simulink model "KakmanFilterSonarExample__Simtestbench"  (R2023b)
settings: Solver=FixedStepAuto  StartTime=0.0  StopTime=Ts*(numel(sonarAlt)-1)  FixedStep=Ts  RelTol=1e-3
undefined symbols (not defined in the file): Discrete, Time, Ts
libraries: simulink x1, ctrlSharedLib x1
settings Model: Creator=leoni  LastModifiedBy=leoni

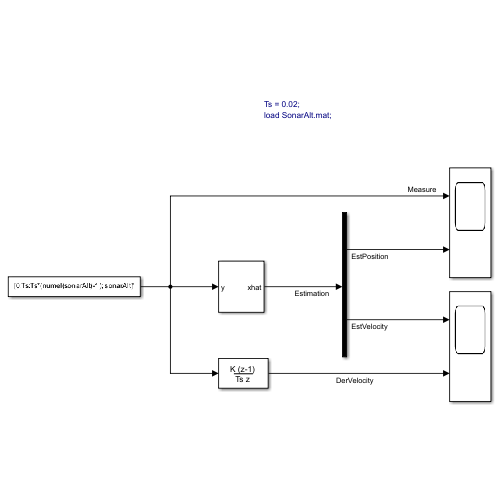
[thumbnail: Simulink's stored preview of the top-level diagram]
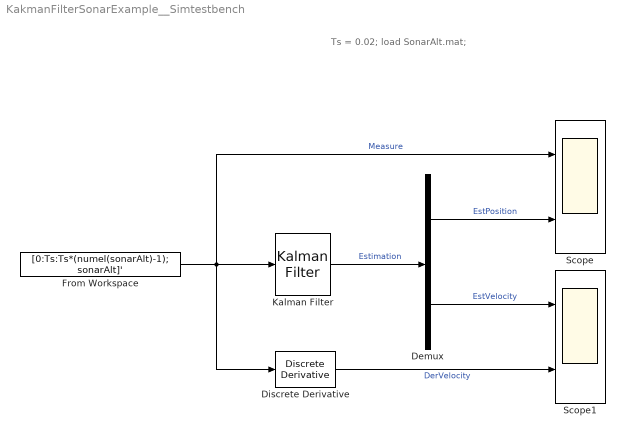
== system KakmanFilterSonarExample__Simtestbench ==
  note: Ts = 0.02;
      | load SonarAlt.mat;
  Demux : Demux  Outputs=2
  Discrete Derivative : simulink/Discrete/Discrete Derivative  gainval=1.0  ICPrevScaledInput=0.0  OutMin=[]  OutMax=[]  OutDataType=fixdt(1, 16)  OutScaling=2^-10  DoSatur=off
  From Workspace : FromWorkspace  VariableName=[0:Ts:Ts*(numel(sonarAlt)-1); sonarAlt]'  SampleTime=Ts
  Kalman Filter : ctrlSharedLib/Kalman Filter  TimeDomain=Discrete-Time  UseCurrentEstimator=on  ModelSource=Individual A, B, C, D matrices  ModelSourceVariable=ss(0.95,1,1,0,1)  A=[1 Ts; 0 1]  B=1  C=[1 0]  D=0  NumberOfStates=1  NumberOfInputs=1  NumberOfOutputs=1  InitialEstimateSource=Dialog  X0=14  P0=10  UseK=off  UseGH=off  NumberOfProcessNoiseInputs=1  G=1  TimeInvariantG=on  H=0  TimeInvariantH=on  Q=[1 0; 0 3]  TimeInvariantQ=on  R=10  TimeInvariantR=on  N=0  TimeInvariantN=on  AddInputPort=off  AddEnablePort=off  OutputEstimatedY=off  OutputP=off  Ts=-1
  Scope : Scope  NumInputPorts=2
  Scope1 : Scope  NumInputPorts=2
  wires:
  From Workspace/1 -> Scope/1, Kalman Filter/1, Discrete Derivative/1  "Measure"
  Kalman Filter/1 -> Demux/1  "Estimation"
  Demux/1 -> Scope/2  "EstPosition"
  Demux/2 -> Scope1/1  "EstVelocity"
  Discrete Derivative/1 -> Scope1/2  "DerVelocity"
